simulink model "SRM_Project"  (R2025b)
settings: Solver=ode4  StartTime=0.0  StopTime=0.2  FixedStep=1e-5  RelTol=1e-3
InitFcn:
  | SRM_params
values from neighbouring files (symbols this model uses):
  TL = out.TorqueData.signals(1).values(:, 2)    [SRM_plots.m]
undefined symbols (not defined in the file or in its folder): B, delta_i, dLdth_vec, Imax, J, L_vec, phase_offset, pole_pitch, Rs, T_max, theta_off, theta_on, theta_ov, theta_vec, tsf_type, Vdc
libraries: slpidlib x1
settings Model: Creator=Dell  LastModifiedBy=adham

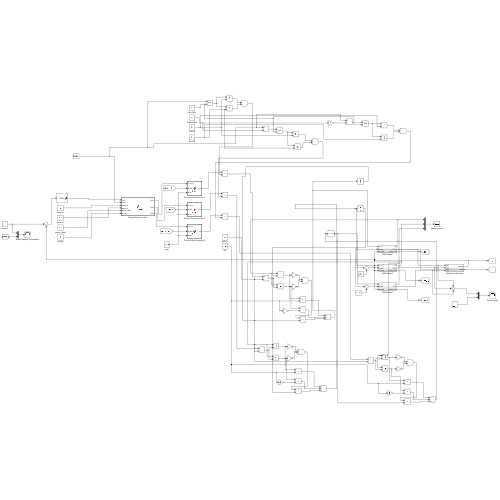
[thumbnail: Simulink's stored preview of the top-level diagram]
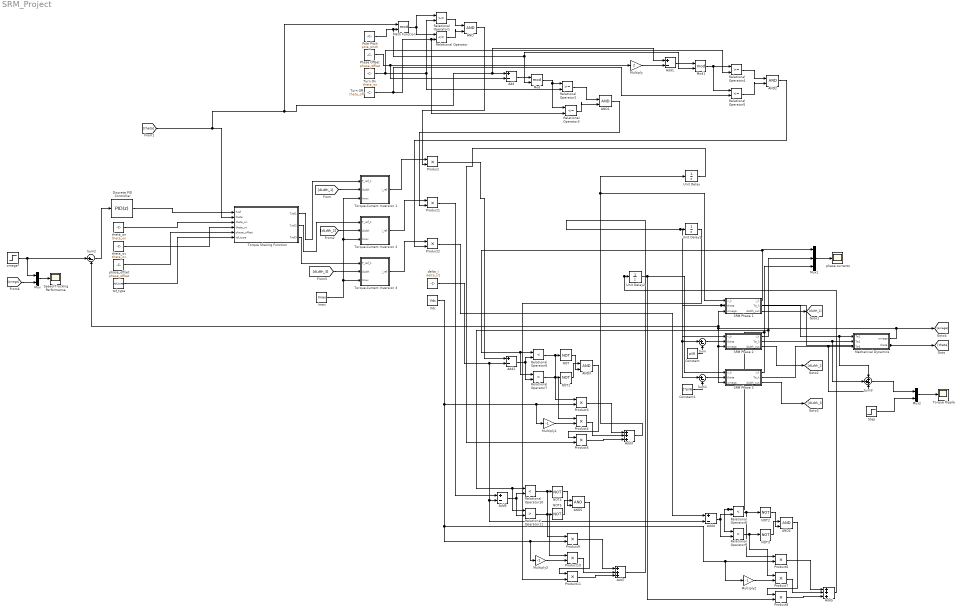
== system SRM_Project ==
  AND{,1..5} (6 alike) : Logic  IconShape=distinctive  AllPortsSameDT=off  OutDataTypeStr=boolean
  Add{,1..2,4,6} (5 alike) : Sum  Inputs=+-
  Add3 : Sum  Inputs=+++
  Add5 : Sum  Inputs=+++
  Add7 : Sum  Inputs=+++
  Constant : Constant  Value=pi/6
  Constant1 : Constant  Value=2*pi/6
  Discrete PID Controller : slpidlib/PID Controller  Controller=PID  Form=Parallel  TimeDomain=Discrete-time  UseExternalTs=off  SampleTime=-1  IntegratorMethod=Forward Euler  FilterMethod=Forward Euler  ControllerParametersSource=internal  P=1  I=1  UseKiTs=off  D=0  UseExternalDerivativeSource=off  N=100  UseFilter=on  TunerSelectOption=Transfer Function Based (PID Tuner App)  InitialConditionSource=internal  InitialConditionForIntegrator=0  InitialConditionForFilter=0  DifferentiatorICPrevScaledInput=0  ExternalReset=none  TrackingMode=off  Kt=1  LimitOutput=on  SatLimitsSource=internal  UpperSaturationLimit=T_max  LowerSaturationLimit=0  LinearizeAsGain=off  AntiWindupMode=none  Kb=1  LimitIntegrator=off  UpperIntegratorSaturationLimit=inf  LowerIntegratorSaturationLimit=-inf  POutMin=[]  POutMax=[]  IOutMin=[]  IOutMax=[]  DOutMin=[]  DOutMax=[]  NOutMin=[]  NOutMax=[]  SumOutMin=[]  SumOutMax=[]  SaturationOutMin=[]  SaturationOutMax=[]  PParamMin=[]  PParamMax=[]  IParamMin=[]  IParamMax=[]  DParamMin=[]  DParamMax=[]  NParamMin=[]  NParamMax=[]  KbParamMin=[]  KbParamMax=[]  KtParamMin=[]  KtParamMax=[]  KbOutMin=[]  KbOutMax=[]  KtOutMin=[]  KtOutMax=[]  IntegratorOutMin=[]  IntegratorOutMax=[]  FilterOutMin=[]  FilterOutMax=[]  SumI1OutMin=[]  SumI1OutMax=[]  SumI2OutMin=[]  SumI2OutMax=[]  SumI3OutMin=[]  SumI3OutMax=[]  SumI4OutMin=[]  SumI4OutMax=[]  SumDOutMin=[]  SumDOutMax=[]  DifferentiatorOutMin=[]  DifferentiatorOutMax=[]  FilterDiffOutCoefMin=[]  FilterDiffOutCoefMax=[]  ReciprocalOutMin=[]  ReciprocalOutMax=[]  SumDenOutMin=[]  SumDenOutMax=[]  SumNumOutMin=[]  SumNumOutMax=[]  DivideOutMin=[]  DivideOutMax=[]  UdiffTsProdOutMin=[]  UdiffTsProdOutMax=[]  NTsProdOutMin=[]  NTsProdOutMax=[]  UintegralTsProdOutMin=[]  UintegralTsProdOutMax=[]  UngainTsProdOutMin=[]  UngainTsProdOutMax=[]  ClampingZeroOutDataTypeStr=Inherit: Inherit via back propagation  ClampingZeroOutMin=[]  ClampingZeroOutMax=[]  FilterDenConstantOutDataTypeStr=Inherit: Inherit via back propagation  FilterDenConstantOutMin=[]  FilterDenConstantOutMax=[]  PCopyOutDataTypeStr=Inherit: Inherit via back propagation  PCopyOutMin=[]  PCopyOutMax=[]  NCopyOutDataTypeStr=Inherit: Inherit via back propagation  NCopyOutMin=[]  NCopyOutMax=[]  IntegratorContinuousStateAttributes=''  IntegratorStateMustResolveToSignalObject=off  IntegratorRTWStateStorageClass=Auto  FilterContinuousStateAttributes=''  FilterStateMustResolveToSignalObject=off  FilterRTWStateStorageClass=Auto  ParallelPVariant=InternalParameters  IdealPVariant=Disabled  IVariant=InternalParameters  DVariant=InternalParameters  IntegratorVariant=Discrete  SatVariant=Enabled  AWVariant=Passthrough  PCopyVariant=Disabled  TRVariant=Disabled  FdbkBlocksVariant=Forward  IdealPFdbkVariant=Disabled  SatFdbkVariant=Disabled  DerivativeFilterVariant=ForwardEulerFilter  NVariant=InternalParameters  NCopyVariant=Disabled  FilterICVariant=InternalICsFilter  IntegratorICVariant=InternalICs  ExternalResetVariant=Disabled  TRSumVariant=Passthrough  SumFdbkVariant=Disabled  SumVariant=Sum_PID  TsampFilterVariant=InternalTs  TsampNgainVariant=Passthrough  TsampIntegralVariant=Disabled_SignalSpec  ExternalSaturationOutDataTypeStr=Inherit: Same as second input  DerivativeSourceVariant=ErrorSignal  PreIntVariant=InternalPreInt
      settings: LibrarySourceBlock=simulink/Discrete/Discrete PID Controller
  Imax : Constant  Value=Imax
  Math Function : Math  Operator=mod
  Mechanical Dynamics : Subsystem
  Mod : Math  Operator=mod
  Mod1 : Math  Operator=mod
  Multiply : Gain  Gain=2
  Multiply1 : Gain  Gain=-1
  Multiply2 : Gain  Gain=-1
  Multiply3 : Gain  Gain=-1
  Mux : Mux  Inputs=2
  Mux1 : Mux  Inputs=3
  Mux2 : Mux  Inputs=2
  NOT{,1..5} (6 alike) : Logic  Operator=NOT  IconShape=distinctive  AllPortsSameDT=off  OutDataTypeStr=boolean
  Phase Offset : Constant  Value=phase_offset
  Pole Pitch : Constant  Value=pole_pitch
  Product{,1..11} (12 alike) : Product
  Relational Operator : RelationalOperator  Operator=<=  OutDataTypeStr=boolean  RndMeth=Simplest  InputSameDT=off
  Relational Operator1 : RelationalOperator  OutDataTypeStr=boolean  RndMeth=Simplest  InputSameDT=off
  Relational Operator10 : RelationalOperator  Operator=<  OutDataTypeStr=boolean  RndMeth=Simplest  InputSameDT=off
  Relational Operator11 : RelationalOperator  Operator=>  OutDataTypeStr=boolean  RndMeth=Simplest  InputSameDT=off
  Relational Operator2 : RelationalOperator  OutDataTypeStr=boolean  RndMeth=Simplest  InputSameDT=off
  Relational Operator3 : RelationalOperator  Operator=<=  OutDataTypeStr=boolean  RndMeth=Simplest  InputSameDT=off
  Relational Operator4 : RelationalOperator  OutDataTypeStr=boolean  RndMeth=Simplest  InputSameDT=off
  Relational Operator5 : RelationalOperator  Operator=<=  OutDataTypeStr=boolean  RndMeth=Simplest  InputSameDT=off
  Relational Operator6 : RelationalOperator  Operator=<  OutDataTypeStr=boolean  RndMeth=Simplest  InputSameDT=off
  Relational Operator7 : RelationalOperator  Operator=>  OutDataTypeStr=boolean  RndMeth=Simplest  InputSameDT=off
  Relational Operator8 : RelationalOperator  Operator=<  OutDataTypeStr=boolean  RndMeth=Simplest  InputSameDT=off
  Relational Operator9 : RelationalOperator  Operator=>  OutDataTypeStr=boolean  RndMeth=Simplest  InputSameDT=off
  SRM Phase 1 : Subsystem
  SRM Phase 2 : Subsystem
  SRM Phase 3 : Subsystem
  Speed-Tracking Performance : Scope
      settings: Title=Speed Tracking Performance  ActiveDisplayYMinimum=78.93066176765771  ActiveDisplayYMaximum=105.87255990529185  YLabel=Omega  DataLoggingVariableName=SpeedData
  Step : Step  Time=0.1  After=TL  SampleTime=0
  Sum : Sum  Inputs=|+-
  Sum1 : Sum  Inputs=|+-
  Sum2 : Sum  Inputs=|+-
  Sum3 : Sum  Inputs=+++
  Torque Ripple : Scope
      settings: ActiveDisplayYMinimum=-0.26462439921975278  ActiveDisplayYMaximum=3.0151430652104114  DataLoggingVariableName=TorqueData
  Torque Sharing Function : MATLAB Function  TreatAsAtomicUnit=on
  Torque-Current Inversion 1 : MATLAB Function  TreatAsAtomicUnit=on
  Torque-Current Inversion 2 : MATLAB Function  TreatAsAtomicUnit=on
  Torque-Current Inversion 3 : MATLAB Function  TreatAsAtomicUnit=on
  Turn Off : Constant  Value=theta_off
  Turn On : Constant  Value=theta_on
  Unit Delay : UnitDelay  SampleTime=-1  HasFrameUpgradeWarning=on
  Unit Delay1 : UnitDelay  SampleTime=-1  HasFrameUpgradeWarning=on
  Unit Delay2 : UnitDelay  SampleTime=-1  HasFrameUpgradeWarning=on
  Vdc : Constant  Value=Vdc
  delta_i : Constant  Value=delta_i/2
  omega* : Step  Time=0  After=100  SampleTime=0
  phase currents : Scope
      settings: ActiveDisplayYMinimum=-0.63560077718964481  ActiveDisplayYMaximum=5.7204069947068081  DataLoggingVariableName=CurrentData
  phase_offset : Constant  Value=phase_offset
  theta_on : Constant  Value=theta_on
  theta_ov : Constant  Value=theta_ov
  tsf_type : Constant  Value=tsf_type
  wires:
  Sum/1 -> SRM Phase 2/2(theta)
  Constant/1 -> Sum/2
  Constant1/1 -> Sum1/2
  Sum1/1 -> SRM Phase 3/2(theta)
  SRM Phase 1/2(Te_k) -> Sum3/1, Mechanical Dynamics/1(Te1)
  SRM Phase 2/2(Te_k) -> Sum3/2, Mechanical Dynamics/2(Te2)
  SRM Phase 3/2(Te_k) -> Sum3/3, Mechanical Dynamics/3(Te3)
  Mechanical Dynamics/1(omega) -> [omega], SRM Phase 1/3(omega), Sum2/2, SRM Phase 3/3(omega), SRM Phase 2/3(omega)
  Mechanical Dynamics/2(theta) -> [theta], Sum/1, Sum1/1, SRM Phase 1/2(theta)
  omega*/1 -> Mux/1, Sum2/1
  Sum2/1 -> Discrete PID Controller/1
  Discrete PID Controller/1 -> Torque Sharing Function/1(Tref)
  Torque Sharing Function/1(Tref1) -> Torque-Current Inversion 1/1(T_ref_k)
  Torque Sharing Function/2(Tref2) -> Torque-Current Inversion 2/1(T_ref_k)
  Torque Sharing Function/3(Tref3) -> Torque-Current Inversion 3/1(T_ref_k)
  Torque-Current Inversion 1/1(i_ref) -> Product/1
  Torque-Current Inversion 2/1(i_ref) -> Product1/1
  Torque-Current Inversion 3/1(i_ref) -> Product2/1
  Product/1 -> Add2/1
  Product1/1 -> Add6/1
  Product2/1 -> Add4/1
  Add3/1 -> Unit Delay/1, SRM Phase 1/1(v_k)
  Add7/1 -> SRM Phase 2/1(v_k), Unit Delay1/1
  Add5/1 -> Unit Delay2/1, Product8/2, SRM Phase 3/1(v_k)
  [theta] -> Torque Sharing Function/2(theta), Math Function/1, Add1/1, Add/1
  SRM Phase 1/1(i_k) -> Relational Operator7/1, Relational Operator6/1, Mux1/1
  SRM Phase 2/1(i_k) -> Mux1/2, Relational Operator11/1, Relational Operator10/1
  SRM Phase 3/1(i_k) -> Mux1/3, Relational Operator9/1, Relational Operator8/1
  theta_on/1 -> Torque Sharing Function/3(theta_on)
  theta_ov/1 -> Torque Sharing Function/4(theta_ov)
  phase_offset/1 -> Torque Sharing Function/5(phase_offset)
  tsf_type/1 -> Torque Sharing Function/6(tsf_type)
  Imax/1 -> Torque-Current Inversion 1/3(Imax), Torque-Current Inversion 2/3(Imax), Torque-Current Inversion 3/3(Imax)
  delta_i/1 -> Add4/2, Add6/2, Add2/2
  Vdc/1 -> Multiply2/1, Product6/2, Multiply3/1, Product9/2, Multiply1/1, Product3/2
  Unit Delay/1 -> Product5/2
  Unit Delay1/1 -> Product11/2
  SRM Phase 1/3(dLdth_out) -> [dLdth_1]
  SRM Phase 2/3(dLdth_out) -> [dLdth_2]
  SRM Phase 3/3(dLdth_out) -> [dLdth_3]
  [dLdth_1] -> Torque-Current Inversion 1/2(dLdth)
  [dLdth_2] -> Torque-Current Inversion 2/2(dLdth)
  [dLdth_3] -> Torque-Current Inversion 3/2(dLdth)
  [omega] -> Mux/2
  Mux/1 -> Speed-Tracking Performance/1
  Mux1/1 -> phase currents/1
  Sum3/1 -> Mux2/1
  Step/1 -> Mux2/2
  Mux2/1 -> Torque Ripple/1
  Pole Pitch/1 -> Mod/2, Mod1/2, Math Function/2
  Math Function/1 -> Relational Operator/1, Relational Operator1/1
  Turn On/1 -> Relational Operator4/2, Relational Operator2/2, Relational Operator1/2
  Turn Off/1 -> Relational Operator5/2, Relational Operator3/2, Relational Operator/2
  Relational Operator1/1 -> AND/1
  Relational Operator/1 -> AND/2
  AND/1 -> Product/2
  Phase Offset/1 -> Add/2, Multiply/1
  Add/1 -> Mod/1
  Mod/1 -> Relational Operator3/1, Relational Operator2/1
  Relational Operator2/1 -> AND1/1
  Relational Operator3/1 -> AND1/2
  AND1/1 -> Product1/2
  Multiply/1 -> Add1/2
  Add1/1 -> Mod1/1
  Mod1/1 -> Relational Operator5/1, Relational Operator4/1
  Relational Operator5/1 -> AND2/2
  Relational Operator4/1 -> AND2/1
  AND2/1 -> Product2/2
  Add2/1 -> Relational Operator7/2, Relational Operator6/2
  Relational Operator6/1 -> Product3/1, NOT/1
  NOT/1 -> AND3/2
  NOT1/1 -> AND3/1
  Relational Operator7/1 -> Product4/1, NOT1/1
  Multiply1/1 -> Product4/2
  AND3/1 -> Product5/1
  Product3/1 -> Add3/1
  Product4/1 -> Add3/2
  Product5/1 -> Add3/3
  Product6/1 -> Add5/1
  Multiply2/1 -> Product7/2
  Relational Operator9/1 -> Product7/1, NOT3/1
  Product8/1 -> Add5/3
  AND4/1 -> Product8/1
  NOT2/1 -> AND4/2
  Add4/1 -> Relational Operator9/2, Relational Operator8/2
  Product7/1 -> Add5/2
  NOT3/1 -> AND4/1
  Relational Operator8/1 -> Product6/1, NOT2/1
  Relational Operator10/1 -> Product9/1, NOT4/1
  Add6/1 -> Relational Operator11/2, Relational Operator10/2
  Product10/1 -> Add7/2
  Product11/1 -> Add7/3
  NOT4/1 -> AND5/2
  NOT5/1 -> AND5/1
  AND5/1 -> Product11/1
  Relational Operator11/1 -> Product10/1, NOT5/1
  Multiply3/1 -> Product10/2
  Product9/1 -> Add7/1

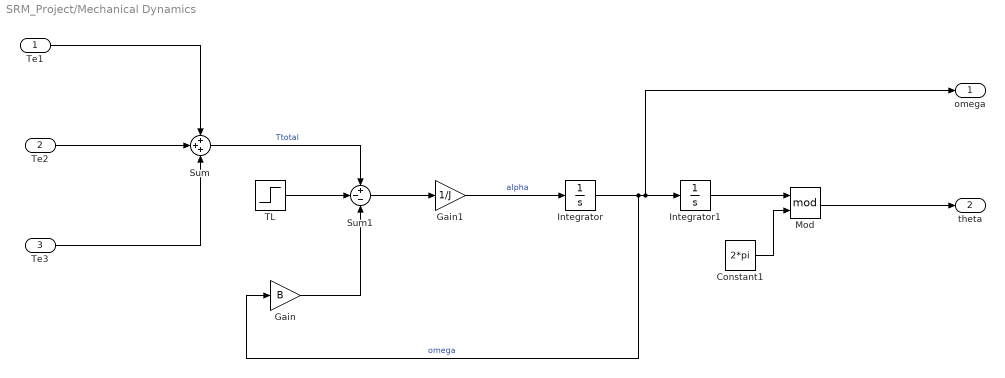
== system SRM_Project/Mechanical Dynamics ==
  Te1 : Inport
  Te2 : Inport  Port=2
  Te3 : Inport  Port=3
  Constant1 : Constant  Value=2*pi
  Gain : Gain  Gain=B
  Gain1 : Gain  Gain=1/J
  Integrator : Integrator
  Integrator1 : Integrator
  Mod : Math  Operator=mod
  Sum : Sum  Inputs=+++
  Sum1 : Sum  Inputs=+--
  TL : Step  Time=0.1  After=TL  SampleTime=0
  omega : Outport
  theta : Outport  Port=2
  wires:
  Te2/1 -> Sum/2
  Te1/1 -> Sum/1
  Te3/1 -> Sum/3
  Sum/1 -> Sum1/1  "Ttotal"
  TL/1 -> Sum1/2
  Gain/1 -> Sum1/3
  Sum1/1 -> Gain1/1
  Gain1/1 -> Integrator/1  "alpha"
  Integrator/1 -> Integrator1/1, omega/1, Gain/1  "omega"
  Integrator1/1 -> Mod/1
  Constant1/1 -> Mod/2
  Mod/1 -> theta/1

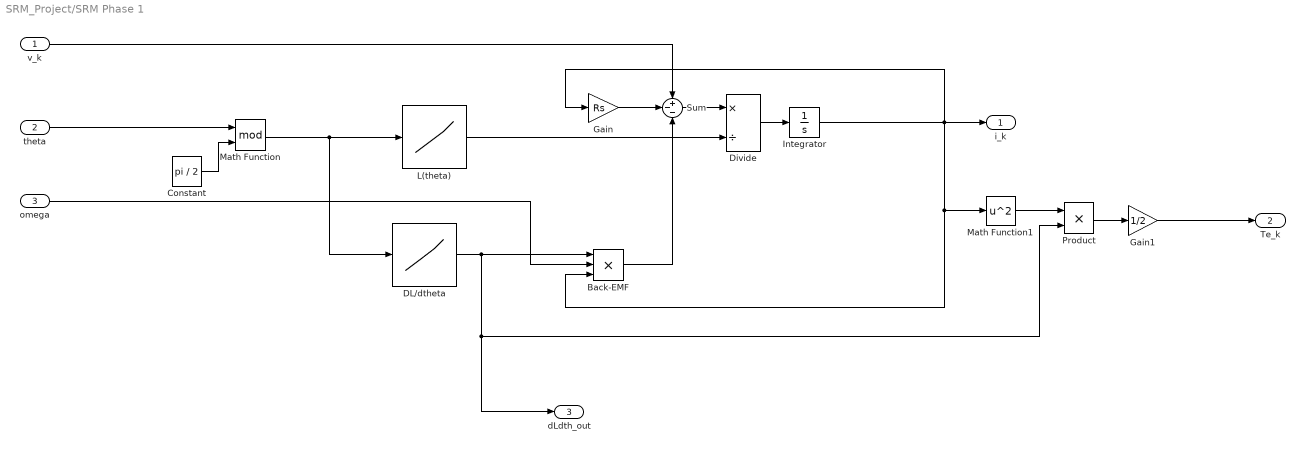
== system SRM_Project/SRM Phase 1 ==
  v_k : Inport
  theta : Inport  Port=2
  omega : Inport  Port=3
  Back-EMF : Product  Inputs=3
  Constant : Constant  Value=pi / 2
  DL/dtheta : Lookup_n-D  NumberOfTableDimensions=1  BreakpointsForDimension1=theta_vec  Table=dLdth_vec  InternalRulePriority=Speed  RndMeth=Simplest
  Divide : Product  Inputs=*/
  Gain : Gain  Gain=Rs
  Gain1 : Gain  Gain=1/2
  Integrator : Integrator  LimitOutput=on  LowerSaturationLimit=0
  L(theta) : Lookup_n-D  NumberOfTableDimensions=1  BreakpointsForDimension1=theta_vec  Table=L_vec  InternalRulePriority=Speed  RndMeth=Simplest
  Math Function : Math  Operator=mod
  Math Function1 : Math  Operator=square
  Product : Product
  Sum : Sum  Inputs=+--
  i_k : Outport
  Te_k : Outport  Port=2
  dLdth_out : Outport  Port=3
  wires:
  theta/1 -> Math Function/1
  Constant/1 -> Math Function/2
  Math Function/1 -> DL/dtheta/1, L(theta)/1
  omega/1 -> Back-EMF/2
  DL/dtheta/1 -> dLdth_out/1, Product/2, Back-EMF/1
  v_k/1 -> Sum/1
  Gain/1 -> Sum/2
  Back-EMF/1 -> Sum/3
  Sum/1 -> Divide/1
  L(theta)/1 -> Divide/2
  Divide/1 -> Integrator/1
  Integrator/1 -> Math Function1/1, Back-EMF/3, i_k/1, Gain/1
  Math Function1/1 -> Product/1
  Product/1 -> Gain1/1
  Gain1/1 -> Te_k/1

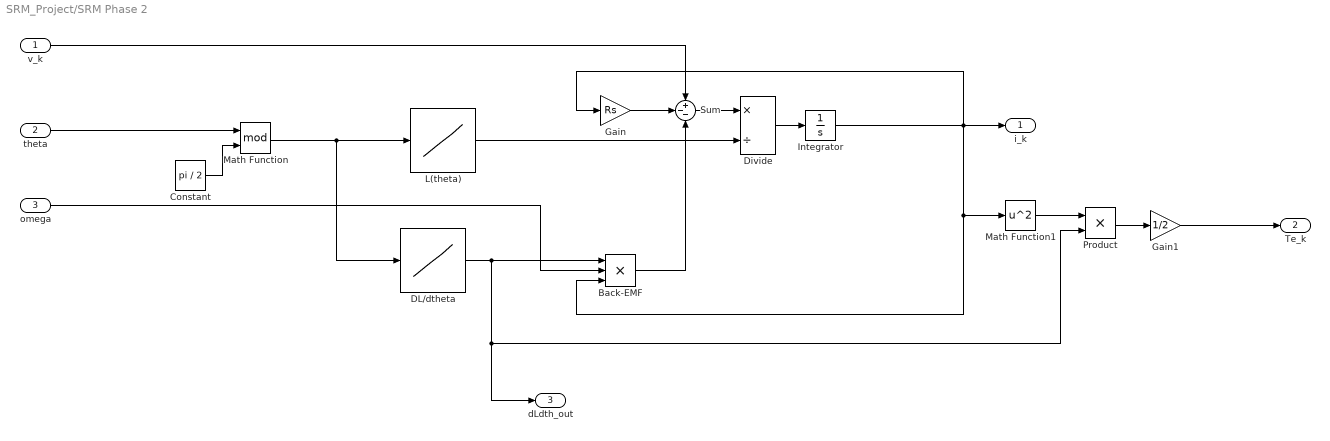
== system SRM_Project/SRM Phase 2 ==
  v_k : Inport
  theta : Inport  Port=2
  omega : Inport  Port=3
  Back-EMF : Product  Inputs=3
  Constant : Constant  Value=pi / 2
  DL/dtheta : Lookup_n-D  NumberOfTableDimensions=1  BreakpointsForDimension1=theta_vec  Table=dLdth_vec  InternalRulePriority=Speed  RndMeth=Simplest
  Divide : Product  Inputs=*/
  Gain : Gain  Gain=Rs
  Gain1 : Gain  Gain=1/2
  Integrator : Integrator  LimitOutput=on  LowerSaturationLimit=0
  L(theta) : Lookup_n-D  NumberOfTableDimensions=1  BreakpointsForDimension1=theta_vec  Table=L_vec  InternalRulePriority=Speed  RndMeth=Simplest
  Math Function : Math  Operator=mod
  Math Function1 : Math  Operator=square
  Product : Product
  Sum : Sum  Inputs=+--
  i_k : Outport
  Te_k : Outport  Port=2
  dLdth_out : Outport  Port=3
  wires:
  theta/1 -> Math Function/1
  Constant/1 -> Math Function/2
  Math Function/1 -> DL/dtheta/1, L(theta)/1
  omega/1 -> Back-EMF/2
  DL/dtheta/1 -> dLdth_out/1, Product/2, Back-EMF/1
  v_k/1 -> Sum/1
  Gain/1 -> Sum/2
  Back-EMF/1 -> Sum/3
  Sum/1 -> Divide/1
  L(theta)/1 -> Divide/2
  Divide/1 -> Integrator/1
  Integrator/1 -> Math Function1/1, Back-EMF/3, i_k/1, Gain/1
  Math Function1/1 -> Product/1
  Product/1 -> Gain1/1
  Gain1/1 -> Te_k/1

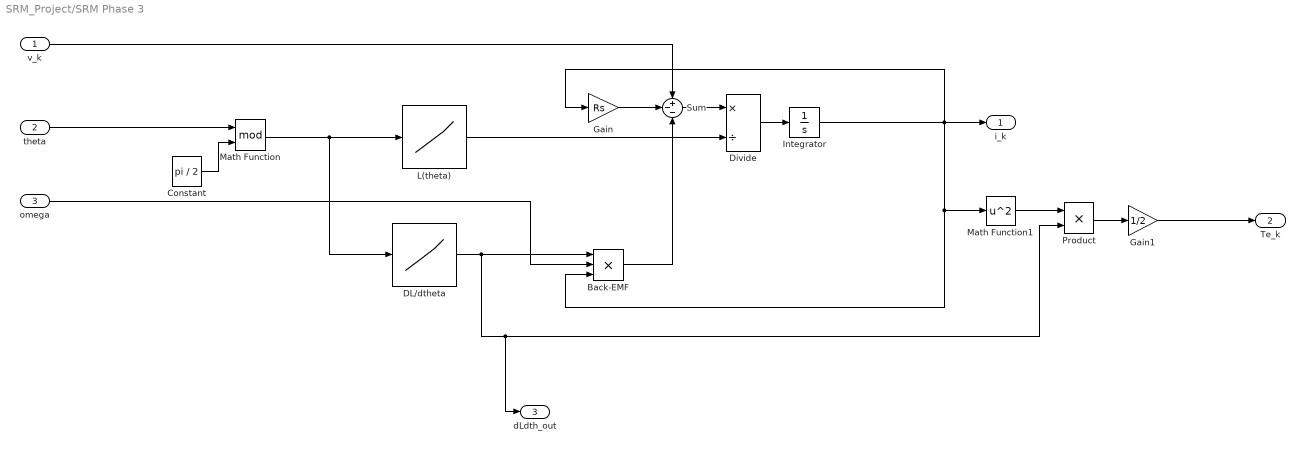
== system SRM_Project/SRM Phase 3 ==
  v_k : Inport
  theta : Inport  Port=2
  omega : Inport  Port=3
  Back-EMF : Product  Inputs=3
  Constant : Constant  Value=pi / 2
  DL/dtheta : Lookup_n-D  NumberOfTableDimensions=1  BreakpointsForDimension1=theta_vec  Table=dLdth_vec  InternalRulePriority=Speed  RndMeth=Simplest
  Divide : Product  Inputs=*/
  Gain : Gain  Gain=Rs
  Gain1 : Gain  Gain=1/2
  Integrator : Integrator  LimitOutput=on  LowerSaturationLimit=0
  L(theta) : Lookup_n-D  NumberOfTableDimensions=1  BreakpointsForDimension1=theta_vec  Table=L_vec  InternalRulePriority=Speed  RndMeth=Simplest
  Math Function : Math  Operator=mod
  Math Function1 : Math  Operator=square
  Product : Product
  Sum : Sum  Inputs=+--
  i_k : Outport
  Te_k : Outport  Port=2
  dLdth_out : Outport  Port=3
  wires:
  theta/1 -> Math Function/1
  Constant/1 -> Math Function/2
  Math Function/1 -> DL/dtheta/1, L(theta)/1
  omega/1 -> Back-EMF/2
  DL/dtheta/1 -> dLdth_out/1, Product/2, Back-EMF/1
  v_k/1 -> Sum/1
  Gain/1 -> Sum/2
  Back-EMF/1 -> Sum/3
  Sum/1 -> Divide/1
  L(theta)/1 -> Divide/2
  Divide/1 -> Integrator/1
  Integrator/1 -> Math Function1/1, Back-EMF/3, i_k/1, Gain/1
  Math Function1/1 -> Product/1
  Product/1 -> Gain1/1
  Gain1/1 -> Te_k/1

== matlab function SRM_Project/Torque Sharing Function ==
  data: Tref input; Tref1 output; theta input; theta_on input; theta_ov input; phase_offset input; tsf_type input; Tref2 output; Tref3 output
function [Tref1, Tref2, Tref3] = TSF_Block(Tref, theta, theta_on, theta_ov, phase_offset, tsf_type)
    pp = pi/2;
    refs = zeros(1,3);
    
    for k = 1:3
        th = mod(theta - (k-1)*phase_offset, pp);
        
        % Rising portion (incoming phase)
        if th >= theta_on && th <= (theta_on + theta_ov)
            x = (th - theta_on)/theta_ov;
            fr = TSF_rising(x, tsf_type);
            refs(k) = fr * Tref;
            
        % Full conduction
        elseif th > (theta_on + theta_ov) && th <= (theta_on + pp/2)
            refs(k) = Tref;
            
        % Falling portion (outgoing phase)
        elseif th > (theta_on + pp/2) && th <= (theta_on + pp/2 + theta_ov)
            x = (th - (theta_on + pp/2))/theta_ov;
            refs(k) = (1 - TSF_rising(x, tsf_type)) * Tref;
            
        else
            refs(k) = 0;
        end
    end
    
    Tref1 = refs(1); Tref2 = refs(2); Tref3 = refs(3);
end

function fr = TSF_rising(x, type)
    switch type
        case 1, fr = x;                           % Linear
        case 2, fr = 0.5*(1 - cos(pi*x));         % Sinusoidal
        case 3, fr = 3*x^2 - 2*x^3;               % Cubic
        case 4, fr = 1 - exp(-3*x);               % Exponential
        otherwise, fr = x;
    end
    fr = min(max(fr, 0), 1); % Bound between 0 and 1
end

== matlab function SRM_Project/Torque-Current Inversion 1 ==
  data: T_ref_k input; i_ref output; dLdth input; Imax input
function i_ref = T_to_I(T_ref_k, dLdth, Imax)
    % 1. Force torque reference to be zero or positive
    T_clean = max(0, T_ref_k);
    
    % 2. Prevent division by zero and get the absolute slope
    slope = max(abs(dLdth), 1e-6);
    
    % 3. The Bulletproof Line: abs() inside the sqrt guarantees 
    % to the Simulink compiler that the output is strictly Real.
    i_ref = sqrt(abs(2 * T_clean / slope));
    
    % 4. Apply hardware limits
    i_ref = min(i_ref, Imax);
end

== matlab function SRM_Project/Torque-Current Inversion 2 ==
  data: T_ref_k input; i_ref output; dLdth input; Imax input
function i_ref = T_to_I(T_ref_k, dLdth, Imax)
    % 1. Force torque reference to be zero or positive
    T_clean = max(0, T_ref_k);
    
    % 2. Prevent division by zero and get the absolute slope
    slope = max(abs(dLdth), 1e-6);
    
    % 3. The Bulletproof Line: abs() inside the sqrt guarantees 
    % to the Simulink compiler that the output is strictly Real.
    i_ref = sqrt(abs(2 * T_clean / slope));
    
    % 4. Apply hardware limits
    i_ref = min(i_ref, Imax);
end

== matlab function SRM_Project/Torque-Current Inversion 3 ==
  data: T_ref_k input; i_ref output; dLdth input; Imax input
function i_ref = T_to_I(T_ref_k, dLdth, Imax)
    % 1. Force torque reference to be zero or positive
    T_clean = max(0, T_ref_k);
    
    % 2. Prevent division by zero and get the absolute slope
    slope = max(abs(dLdth), 1e-6);
    
    % 3. The Bulletproof Line: abs() inside the sqrt guarantees 
    % to the Simulink compiler that the output is strictly Real.
    i_ref = sqrt(abs(2 * T_clean / slope));
    
    % 4. Apply hardware limits
    i_ref = min(i_ref, Imax);
end
